simulink model "Induction_motor_simulink_model"  (R2023b)
settings: Solver=ode23t  StartTime=0.0  StopTime=5  MaxStep=1e-4  RelTol=1e-3
libraries: eeRmsMeasurement x7, spsSeriesRLCBranchLib x4, spsThreePhaseBreakerLib x2, spsAsynchronousMachineSIUnitsLib x1, spsPower3phInstantaneousLib x1, simulink x1, spsThreePhaseVIMeasurementLib x1, spsThreePhaseFaultLib x1, spsThreePhaseSourceLib x1, spsUniversalBridgeLib x1, spspowerguiLib x1
settings Model: Creator=DSP & Communication  LastModifiedBy=PMYLS
settings DebuggingCC: UnconnectedInputMsg=warning  UnconnectedOutputMsg=warning  UnconnectedLineMsg=warning
settings ModelReferenceCC: EnableRefExpFcnMdlSchedulingChecks=on
settings RTWCC: DLArmComputeVersion=19.05

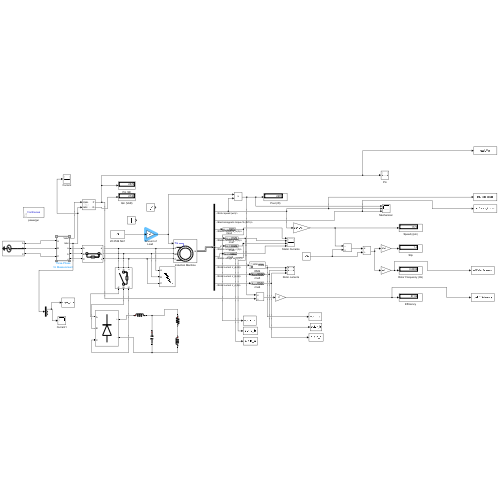
[thumbnail: Simulink's stored preview of the top-level diagram]
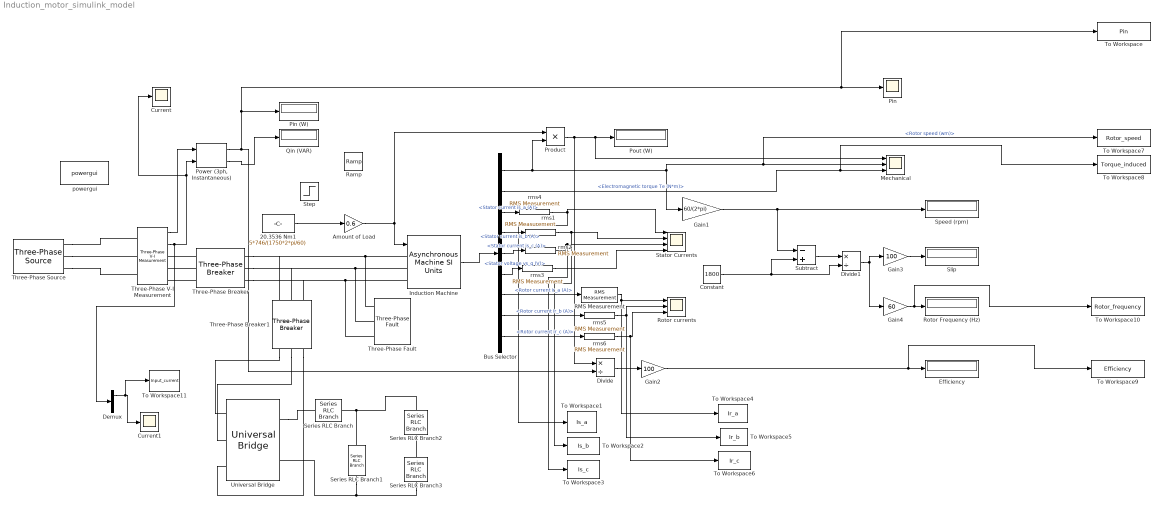
== system Induction_motor_simulink_model ==
  20.3536 Nm1 : Constant  Value=5*746/(1750*2*pi/60)
  "Amount of Load " : Gain  Gain=0.6
  Bus Selector : BusSelector  OutputSignals=Mechanical.Rotor speed (wm),Mechanical.Electromagnetic torque Te (N*m),Stator measurements.Stator current is_a (A),Stator measurements.Stator current is_b (A),Stator measurements.Stator current is_c (A),Stator measurements.Stator voltage vs_q (V),Rotor measurements.Rotor current ir_a (A),Rotor measurements.Rotor current ir_b (A),Rotor measurements.Rotor current ir_c (A)
  Constant : Constant  Value=1800
  Current : Scope
  Current1 : Scope
  Demux : Demux  Outputs=3
  Divide : Product  Inputs=*/
  Divide1 : Product  Inputs=*/
  Efficiency : Display
  Gain1 : Gain  Gain=60/(2*pi)
  Gain2 : Gain  Gain=100
  Gain3 : Gain  Gain=100
  Gain4 : Gain  Gain=60
  "Induction Machine " : spsAsynchronousMachineSIUnitsLib/Asynchronous Machine SI Units  RotorType=Squirrel-cage  PresetModel="01:  5 HP   460 V 60Hz 1750 RPM"  MechanicalLoad=Torque Tm  ShowDetailedParameters=on  ReferenceFrame=Rotor  Units=SI  MeasurementBus=off  NominalParameters=[3730 460 60]  VoltageRatio=1  Stator=[1.115 0.005974]  Rotor=[1.083 0.005974]  Cage1=[0.4155 0.002066]  Cage2=[0.4168 0.0003495]  Lm=0.2037  Mechanical=[0.02 0.005752 2]  PolePairs=2  InitialConditions=[0 0 0 0 0 0 0 0]  SimulateSaturation=off  Saturation=[14.03593122, 27.81365428, 53.79336849, 72.68890987, 97.98006896, 148.6815601, 215.7428561, 302.9841135, 428.7778367 ; 230, 322, 414, 460, 506, 552, 598, 644, 690]  LoadFlowParameters=1492000  TsPowergui=0  TsBlock=-1  IterativeModel=Trapezoidal non iterative  IterativeDiscreteModel=Trapezoidal non iterative  Pmec=1.492e+006
  "Mechanical " : Scope  NumInputPorts=3
  Pin : Scope
  Pin (W) : Display
  Pout (W) : Display
  "Power (3ph, Instantaneous)" : spsPower3phInstantaneousLib/Power (3ph, Instantaneous)
  Product : Product
  Qin (VAR) : Display
  RMS Measurement : eeRmsMeasurement/RMS Measurement  LabelModeActiveChoice=Total  F=60  SpecifyHarmonics=off  K=[0 1 2]  Ts=0
      settings: LibrarySourceBlock=|
      | ee_sl_lib/Measurements/RMS
      | Measurement
  Ramp : simulink/Sources/Ramp  slope=10  start=2  InitialOutput=5*746/(1750*2*pi/60)
  Rotor Frequency (Hz) : Display
  Rotor currents : Scope  NumInputPorts=3
  Series RLC Branch : spsSeriesRLCBranchLib/Series RLC Branch  LConnTagsString=__new0  RConnTagsString=__new0  BranchType=L  Resistance=1  Inductance=1e-3  SetiL0=off  InitialCurrent=0  Capacitance=1e-6  Setx0=off  InitialVoltage=0  Measurements=None
  Series RLC Branch1 : spsSeriesRLCBranchLib/Series RLC Branch  LConnTagsString=__new0  RConnTagsString=__new0  BranchType=C  Resistance=1  Inductance=1e-3  SetiL0=off  InitialCurrent=0  Capacitance=10e-6  Setx0=off  InitialVoltage=0  Measurements=None
  Series RLC Branch2 : spsSeriesRLCBranchLib/Series RLC Branch  LConnTagsString=__new0  RConnTagsString=__new0  BranchType=R  Resistance=100  Inductance=1e-3  SetiL0=off  InitialCurrent=0  Capacitance=1e-6  Setx0=off  InitialVoltage=0  Measurements=None
  Series RLC Branch3 : spsSeriesRLCBranchLib/Series RLC Branch  LConnTagsString=__new0  RConnTagsString=__new0  BranchType=L  Resistance=1  Inductance=1e-3  SetiL0=off  InitialCurrent=0  Capacitance=1e-6  Setx0=off  InitialVoltage=0  Measurements=None
  Slip : Display
  Speed (rpm) : Display
  Stator Currents : Scope  NumInputPorts=4
  Step : Step  Time=3  Before=5*746/(1750*2*pi/60)  After=3*5*746/(1750*2*pi/60)  SampleTime=0
  Subtract : Sum  Inputs=-+
  Three-Phase V-I Measurement : spsThreePhaseVIMeasurementLib/Three-Phase V-I Measurement  VoltageMeasurement=phase-to-ground  SetLabelV=off  LabelV=Vabc  Vpu=off  VpuLL=off  CurrentMeasurement=yes  SetLabelI=off  LabelI=Iabc  Ipu=off  Pbase=100e6  Vbase=500e3  OutputType=Complex  PhasorSimulation=off  PSBequivalent=0
  Three-Phase Breaker : spsThreePhaseBreakerLib/Three-Phase Breaker  InitialState=closed  SwitchA=off  SwitchB=off  SwitchC=off  SwitchTimes="[2  5]"  External=off  BreakerResistance=0.01  SnubberResistance=1e6  SnubberCapacitance=inf  Measurements=None
  Three-Phase Breaker1 : spsThreePhaseBreakerLib/Three-Phase Breaker  InitialState=open  SwitchA=off  SwitchB=off  SwitchC=off  SwitchTimes=[3 5]  External=off  BreakerResistance=0.01  SnubberResistance=1e6  SnubberCapacitance=inf  Measurements=None
  Three-Phase Fault : spsThreePhaseFaultLib/Three-Phase Fault  InitialStates=0  FaultA=off  FaultB=off  FaultC=off  GroundFault=off  SwitchTimes="[2  5]"  External=off  SwitchStatus=NaN  FaultResistance=0.01  GroundResistance=0.001  SnubberResistance=1e6  SnubberCapacitance=inf  Measurements=None
  Three-Phase Source : spsThreePhaseSourceLib/Three-Phase Source  InternalConnection=Yg  VoltagePhases=off  Voltage=460  PhaseAngle=0  Voltage_phases=[25e3 25e3 25e3]/sqrt(3)  PhaseAngles_phases=[0 -120 +120]  Frequency=60  NonIdealSource=off  SpecifyImpedance=off  Resistance=0.8929  Inductance=16.58e-3  ShortCircuitLevel=100e6  BaseVoltage=25e3  XRratio=7  BusType=swing  Pref=10e3  Qref=0  Prefabc=[10e3, 10e3, 10e3]  Qrefabc=[0, 0, 0]  Qmin=-inf  Qmax=inf
  To Workspace : ToWorkspace  VariableName=Pin  SampleTime=-1
      settings: MaxDataPoints=10000  Save2DSignal=2-D array (concatenate along first dimension)
  To Workspace1 : ToWorkspace  VariableName=Is_a  SampleTime=-1
      settings: MaxDataPoints=10000  Save2DSignal=2-D array (concatenate along first dimension)
  To Workspace10 : ToWorkspace  VariableName=Rotor_frequency  SampleTime=-1
      settings: MaxDataPoints=10000  Save2DSignal=2-D array (concatenate along first dimension)
  To Workspace11 : ToWorkspace  VariableName=Input_current  SampleTime=-1
      settings: MaxDataPoints=10000  Save2DSignal=2-D array (concatenate along first dimension)
  To Workspace2 : ToWorkspace  VariableName=Is_b  SampleTime=-1
      settings: MaxDataPoints=10000  Save2DSignal=2-D array (concatenate along first dimension)
  To Workspace3 : ToWorkspace  VariableName=Is_c  SampleTime=-1
      settings: MaxDataPoints=10000  Save2DSignal=2-D array (concatenate along first dimension)
  To Workspace4 : ToWorkspace  VariableName=Ir_a  SampleTime=-1
      settings: MaxDataPoints=10000  Save2DSignal=2-D array (concatenate along first dimension)
  To Workspace5 : ToWorkspace  VariableName=Ir_b  SampleTime=-1
      settings: MaxDataPoints=10000  Save2DSignal=2-D array (concatenate along first dimension)
  To Workspace6 : ToWorkspace  VariableName=Ir_c  SampleTime=-1
      settings: MaxDataPoints=10000  Save2DSignal=2-D array (concatenate along first dimension)
  To Workspace7 : ToWorkspace  VariableName=Rotor_speed  SampleTime=-1
      settings: MaxDataPoints=10000  Save2DSignal=2-D array (concatenate along first dimension)
  To Workspace8 : ToWorkspace  VariableName=Torque_induced  SampleTime=-1
      settings: MaxDataPoints=10000  Save2DSignal=2-D array (concatenate along first dimension)
  To Workspace9 : ToWorkspace  VariableName=Efficiency  SampleTime=-1
      settings: MaxDataPoints=10000  Save2DSignal=2-D array (concatenate along first dimension)
  Universal Bridge : spsUniversalBridgeLib/Universal Bridge  Arms=3  SnubberResistance=1e5  SnubberCapacitance=inf  Device=Diodes  Ron=1e-3  Lon=0  ForwardVoltages="[  0  0  ]"  ForwardVoltage=0  GTOparameters=[ 10e-6 , 20e-6 ]  IGBTparameters=[ 1e-6 , 2e-6 ]  Measurements=None  Measurements_2=None  converterType=Rectifier
  powergui : spspowerguiLib/powergui  Priority=1  SimulationMode=Continuous  SampleTime=50e-6  frequency=60  Iterations=50  frequencyindice=60  Pbase=100e6  ErrMax=1e-4  UnitsV=kV  UnitsW=MW  buscounter=0  FunctionMessages=off  echomessages=off  EnableUseOfTLC=off  CurrentSourceSwitches=off  DisableSnubberDevices=off  DisableRonSwitches=off  DisableVfSwitches=off  DisplayEquations=off  AutomaticDiscreteSolvers=off  SolverType=Tustin/Backward Euler (TBE)  Interpol=off  ExternalGateDelay=off  methode=off  Ts=100  x0status=blocks  SPID=on  SwTol=0  HookPort=off  NonlinearTolerance=1e-4  nMaxIteration=100  ContinueOnMaxIteration=off  RestoreLinks=warning  ResistiveCurrentMeasurement=off  Frange=[0:2:500]  Ylog=off  Xlog=on  ShowGrid=off  save=off  variable=ZData  structure=0  ZoomFFT=off  StartTime=0.0  cycles=1  DisplayStyle=1  fundamental=60  FreqAxis=off  MaxFrequency=1000  frequencyindicesteady=1  RmsSteady=1  display=off
  rms{1..6} (6 alike) : eeRmsMeasurement/RMS Measurement  LabelModeActiveChoice=Total  F=60  SpecifyHarmonics=off  K=[0 1 2]  Ts=0
      settings: LibrarySourceBlock=|
      | ee_sl_lib/Measurements/RMS
      | Measurement
  wires:
  "Induction Machine "/1 -> Bus Selector/1
  "Amount of Load "/1 -> "Induction Machine "/1, Product/1
  Three-Phase V-I Measurement/1 -> "Power (3ph, Instantaneous)"/1
  Three-Phase V-I Measurement/2 -> Demux/1, Current/1, "Power (3ph, Instantaneous)"/2
  "Power (3ph, Instantaneous)"/1 -> Divide/2, To Workspace/1, Pin/1, Pin (W)/1
  Gain1/1 -> Subtract/1, Speed (rpm)/1
  Bus Selector/1 -> Gain1/1, To Workspace7/1, "Mechanical "/2, Product/2  "<Rotor speed (wm)>"
  Product/1 -> "Mechanical "/1, Pout (W)/1, Divide/1
  "Power (3ph, Instantaneous)"/2 -> Qin (VAR)/1
  Bus Selector/2 -> To Workspace8/1, "Mechanical "/3  "<Electromagnetic torque Te (N*m)>"
  Bus Selector/3 -> rms4/1  "<Stator current is_a (A)>"
  Bus Selector/4 -> rms1/1  "<Stator current is_b (A)>"
  Bus Selector/5 -> rms2/1  "<Stator current is_c (A)>"
  Bus Selector/7 -> RMS Measurement/1  "<Rotor current ir_a (A)>"
  Bus Selector/8 -> rms5/1  "<Rotor current ir_b (A)>"
  Bus Selector/9 -> rms6/1  "<Rotor current ir_c (A)>"
  Bus Selector/6 -> rms3/1  "<Stator voltage vs_q (V)>"
  Divide/1 -> Gain2/1
  Gain2/1 -> To Workspace9/1, Efficiency/1
  Gain3/1 -> Slip/1
  Constant/1 -> Subtract/2, Divide1/2
  Subtract/1 -> Divide1/1
  Divide1/1 -> Gain3/1, Gain4/1
  Gain4/1 -> To Workspace10/1, Rotor Frequency (Hz)/1
  rms1/1 -> To Workspace2/1, Stator Currents/2
  rms2/1 -> To Workspace3/1, Stator Currents/3
  rms3/1 -> Stator Currents/4
  RMS Measurement/1 -> To Workspace4/1, Rotor currents/1
  rms5/1 -> Rotor currents/2, To Workspace5/1
  rms6/1 -> To Workspace6/1, Rotor currents/3
  rms4/1 -> Stator Currents/1, To Workspace1/1
  Demux/1 -> To Workspace11/1, Current1/1
  20.3536 Nm1/1 -> "Amount of Load "/1
  connections:
  Three-Phase Fault/LConn3 -- Three-Phase Breaker1/RConn3 -- Three-Phase Breaker/RConn3 -- "Induction Machine "/LConn3
  Three-Phase Fault/LConn2 -- Three-Phase Breaker1/RConn2 -- Three-Phase Breaker/RConn2 -- "Induction Machine "/LConn2
  Three-Phase Fault/LConn1 -- Three-Phase Breaker1/RConn1 -- Three-Phase Breaker/RConn1 -- "Induction Machine "/LConn1
  Three-Phase Source/RConn1 -- Three-Phase V-I Measurement/LConn1
  Three-Phase Source/RConn2 -- Three-Phase V-I Measurement/LConn2
  Three-Phase Source/RConn3 -- Three-Phase V-I Measurement/LConn3
  Three-Phase Breaker/LConn1 -- Three-Phase V-I Measurement/RConn1
  Three-Phase Breaker/LConn2 -- Three-Phase V-I Measurement/RConn2
  Three-Phase Breaker/LConn3 -- Three-Phase V-I Measurement/RConn3
  Universal Bridge/RConn1 -- Series RLC Branch/LConn1
  Series RLC Branch3/LConn1 -- Series RLC Branch2/RConn1
  Series RLC Branch1/LConn1 -- Series RLC Branch/RConn1 -- Series RLC Branch2/LConn1
  Series RLC Branch3/RConn1 -- Series RLC Branch1/RConn1 -- Universal Bridge/RConn2
  Three-Phase Breaker1/LConn1 -- Universal Bridge/LConn1
  Three-Phase Breaker1/LConn2 -- Universal Bridge/LConn2
  Three-Phase Breaker1/LConn3 -- Universal Bridge/LConn3
